simulink model "PrinterILC_sim"  (Simulink 7.8)
settings: Solver=FixedStepDiscrete  StartTime=0.0  StopTime=5  FixedStep=1/1000  RelTol=1e-3
libraries: simulink x2, cstblocks x1
settings Model: Creator=jbolder  LastModifiedBy=JZundert
settings CodeAppCC: CustomSymbolStrType=$N$R$M_T
settings GRTTargetCC: TargetFunctionLibrary=C89/C90 (ANSI)

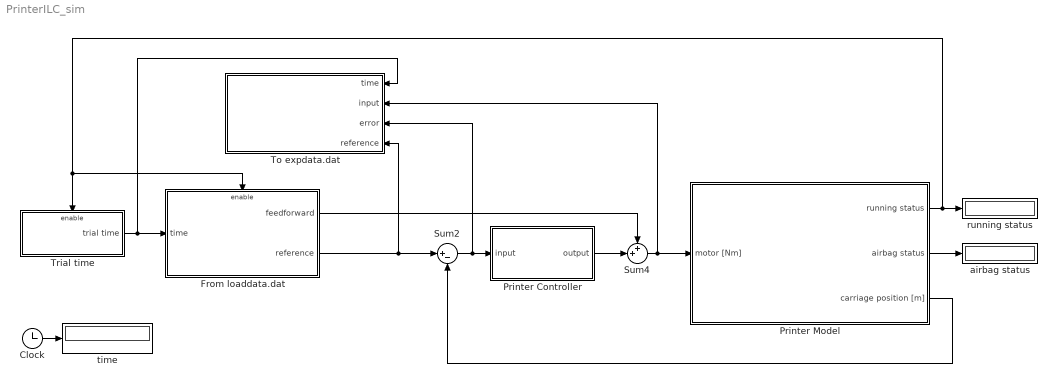
== system PrinterILC_sim ==
  Clock : Clock
  From loaddata.dat : Subsystem
  Printer Controller : Subsystem
  Printer Model : Subsystem  InitFcn=load('PrinterModel.mat');
  Sum2 : Sum  Inputs=|+-
  Sum4 : Sum  Inputs=++|  SaturateOnIntegerOverflow=on  InputSameDT=on  OutDataTypeStr=Inherit: Same as first input
  To expdata.dat : Subsystem
  Trial time : Subsystem  TreatAsAtomicUnit=on
  airbag status : Display
      settings: Decimation=50
  running status : Display
      settings: Decimation=50
  time : Display
      settings: Decimation=50
  wires:
  Sum2/1 -> To expdata.dat/3(error), Printer Controller/1(input)
  From loaddata.dat/2(reference) -> Sum2/1, To expdata.dat/4(reference)
  Clock/1 -> time/1
  Printer Model/3(carriage position [m]) -> Sum2/2
  Printer Controller/1(output) -> Sum4/2
  From loaddata.dat/1(feedforward) -> Sum4/1
  Sum4/1 -> Printer Model/1(motor [Nm]), To expdata.dat/2(input)
  Printer Model/1(running status) -> running status/1, Trial time/Enable, From loaddata.dat/Enable
  Trial time/1(trial time) -> From loaddata.dat/1(time), To expdata.dat/1(time)
  Printer Model/2(airbag status) -> airbag status/1

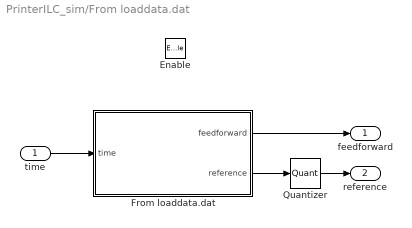
== system PrinterILC_sim/From loaddata.dat ==
  time : Inport
  Enable : EnablePort  StatesWhenEnabling=reset
  From loaddata.dat : Subsystem
  Quantizer : Quantizer  QuantizationInterval=1/(600*100/2.54)
  feedforward : Outport
  reference : Outport  Port=2
  wires:
  time/1 -> From loaddata.dat/1(time)
  From loaddata.dat/1(feedforward) -> feedforward/1
  From loaddata.dat/2(reference) -> Quantizer/1
  Quantizer/1 -> reference/1

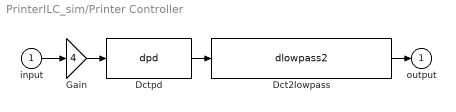
== system PrinterILC_sim/Printer Controller ==
  input : Inport
  Dct2lowpass : S-Function  FunctionName=dlowpass2  Parameters=f_den, b_den, 0.001  EnableBusSupport=off  mask(dctools){f_den=40, b_den=0.7}
      mask prompts: f_den "Pole [Hz]"; b_den "Damping pole [-]"
      mask help: This block implements a discrete time 2nd order lowpass filter.
      mask Display: disp('DCT 2nd order lowpass')
  Dctpd : S-Function  FunctionName=dpd  Parameters=kp, kv, 0.001  EnableBusSupport=off  mask(dctools){kp=40, kv=1}
      mask help: This block implements a discrete time pd filter.
      mask Display: disp('DCT pd')
  Gain : Gain  Gain=4  SaturateOnIntegerOverflow=on  OutDataTypeStr=Inherit: Same as input  ParamDataTypeStr=Inherit: Same as input
  output : Outport
  wires:
  input/1 -> Gain/1
  Gain/1 -> Dctpd/1
  Dctpd/1 -> Dct2lowpass/1
  Dct2lowpass/1 -> output/1

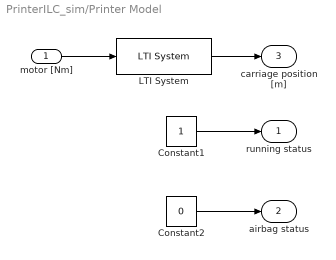
== system PrinterILC_sim/Printer Model ==
  motor [Nm] : Inport
  Constant1 : Constant
  Constant2 : Constant  Value=0
  LTI System : cstblocks/LTI System  sys=PrinterModelSS  IC=[]
  running status : Outport
  airbag status : Outport  Port=2
  carriage position [m] : Outport  Port=3
  wires:
  Constant1/1 -> running status/1
  Constant2/1 -> airbag status/1
  motor [Nm]/1 -> LTI System/1
  LTI System/1 -> carriage position [m]/1

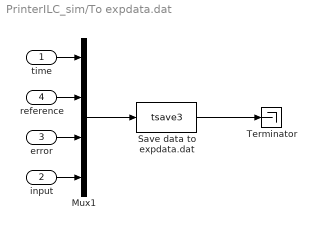
== system PrinterILC_sim/To expdata.dat ==
  time : Inport
  input : Inport  Port=2
  error : Inport  Port=3
  reference : Inport  Port=4
  Mux1 : Mux
  Save data to expdata.dat : S-Function  FunctionName=tsave3  Parameters=0  EnableBusSupport=off
  Terminator : Terminator
  wires:
  Mux1/1 -> Save data to expdata.dat/1
  Save data to expdata.dat/1 -> Terminator/1
  time/1 -> Mux1/1
  input/1 -> Mux1/4
  error/1 -> Mux1/3
  reference/1 -> Mux1/2

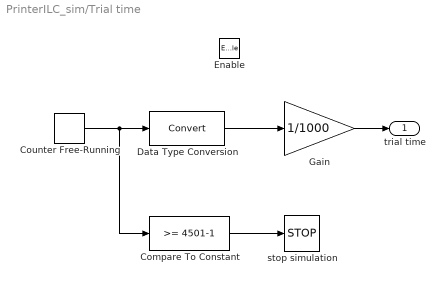
== system PrinterILC_sim/Trial time ==
  Enable : EnablePort  StatesWhenEnabling=reset
  Compare To Constant : simulink/Logic and Bit Operations/Compare To Constant  relop=>=  const=4501-1  OutDataTypeStr=boolean
  Counter Free-Running : simulink/Sources/Counter Free-Running  NumBits=32  tsamp=-1
  Data Type Conversion : DataTypeConversion
  Gain : Gain  Gain=1/1000
  stop simulation : Stop
  trial time : Outport  InitialOutput=0
  wires:
  Counter Free-Running/1 -> Compare To Constant/1, Data Type Conversion/1
  Compare To Constant/1 -> stop simulation/1
  Data Type Conversion/1 -> Gain/1
  Gain/1 -> trial time/1

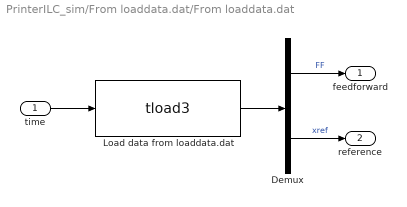
== system PrinterILC_sim/From loaddata.dat/From loaddata.dat ==
  time : Inport
  Demux : Demux  Outputs=2
  Load data from loaddata.dat : S-Function  FunctionName=tload3  Parameters=0  EnableBusSupport=off
  feedforward : Outport
  reference : Outport  Port=2
  wires:
  time/1 -> Load data from loaddata.dat/1
  Load data from loaddata.dat/1 -> Demux/1
  Demux/1 -> feedforward/1  "FF"
  Demux/2 -> reference/1  "xref"
